simulink model "Chapter_9_Section_6_Model"  (R2019b)
settings: Solver=FixedStepAuto  StartTime=0.0  StopTime=500  FixedStep=0.02  RelTol=1e-3  EnableMultiTasking=on
libraries: arduinolib x1, simulink x1
settings Model: SimulationMode=external  ExtModeTrigDuration=2  Creator=nbibin001  LastModifiedBy=covasanvictor
settings DataIOCC: ReturnWorkspaceOutputs=off
settings OptimizationCC: PassReuseOutputArgsAs=Individual arguments  MaxStackSize=64  EfficientTunableParamExpr=on
settings DebuggingCC: ParameterTunabilityLossMsg=error  ArithmeticOperatorsInVariantConditions=warning
settings HardwareCC: ProdBitPerInt=16  ProdBitPerPointer=16  ProdBitPerSizeT=16  ProdBitPerPtrDiffT=16  ProdLargestAtomicFloat=None  ProdWordSize=8  ProdHWDeviceType=Atmel->AVR
settings SFSimCC: SimUseLocalCustomCode=off  MATLABDynamicMemAlloc=off  CustomCodeUndefinedFunction=UseInterfaceOnly
settings RTWCC: SystemTargetFile=ert.tlc  HardwareBoard=Arduino Mega 2560  TLCOptions=-aInlineSetEventsForThisBaseRateFcn=TLC_FALSE -aSuppressMultiTaskScheduler=TLC_FALSE -aRateBasedStepFcn=1  TemplateMakefile=ert_default_tmf  GenerateReport=on  RTWUseLocalCustomCode=off  Toolchain=Arduino AVR  BuildConfiguration=Faster Runs  IncludeHyperlinkInReport=on  LaunchReport=on  GenerateTraceInfo=on  GenerateTraceReport=on  GenerateTraceReportSl=on  GenerateTraceReportSf=on  GenerateTraceReportEml=on
settings CodeAppCC: ForceParamTrailComments=on  IgnoreCustomStorageClasses=off  OperatorAnnotations=on  SimulinkDataObjDesc=on  SFDataObjDesc=on  MATLABFcnDesc=on  InsertBlockDesc=on  StateflowObjectComments=on  MATLABSourceComments=on
settings ERTTargetCC: SupportContinuousTime=on  SupportVariableSizeSignals=on

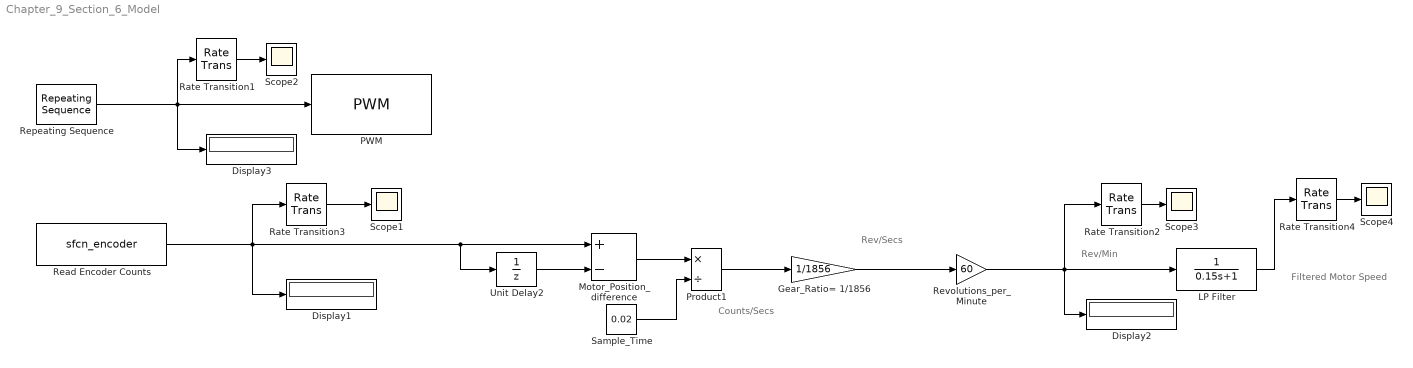
== system Chapter_9_Section_6_Model ==
  note: Counts/Secs
  note: Rev/Secs
  note: Rev/Min
  note: Filtered Motor Speed
  Display1 : Display
  Display2 : Display
  Display3 : Display
  Gear_Ratio= 1/1856 : Gain  Gain=1/1856
  LP Filter : TransferFcn  Denominator=[0.15 1]
  Motor_Position_difference : Sum  Inputs=+-
  PWM : arduinolib/PWM  pinNumber=5  EnableInputFrequency=off  InitialFrequency=2000  InitialDutyCycle=0  NotificationType=None  blockPlatform=arduino
  Product1 : Product  Inputs=*/
  Rate Transition{1..4} (4 alike) : RateTransition
  Read Encoder Counts : S-Function  InitFcn=try, set_param(gcb,'FunctionName','sfcn_encoder'), end  FunctionName=sfcn_encoder  Parameters=uint8(0),uint8(2),uint8(3)  SFunctionModules=sfcn_encoder_wrapper  SFunctionDeploymentMode=off  EnableBusSupport=off  mask(S-Function Builder){}
      mask init:
      | val = [[.9  0.75 0.75 1 1 .9 .9 1]',[1 1 0.75 0.75 .9 .9 1 .9]'];try , sys = get_param(gcb,'SfunBuilderFcnName');if isempty(sys), sys = get_param(gcb,'FunctionName'); end,catch, sys = get_param(gcb,'FunctionName'); end
      settings: CopyFcn=set_param(gcbh,'LinkStatus','none')  PreSaveFcn=try, set_param(gcb,'FunctionName','sfcn_encoder'), end  OpenFcn=sfunctionwizard(gcbh)
      mask Display: plot(val(:,1),val(:,2)),disp(sys), port_label('output',1,'pos')
  Repeating Sequence : simulink/Sources/Repeating Sequence  rep_seq_t="[0 \t  49.9   50   99.9 100  149.9  150 199.9 \t200   249.9   250 299.9 300   349.9   350 399.9 400   449.9   450 500]"  rep_seq_y="[25.5 25.5   50.1 50.1 76.5 76.5   102 102\t    127.5 127.5   153 153   178.5 178.5   204 204   229.5 229.5   255 255]"
  Revolutions_per_Minute : Gain  Gain=60
  Sample_Time : Constant  Value=0.02
  Scope{1..4} (4 alike) : Scope
  Unit Delay2 : UnitDelay  SampleTime=-1  HasFrameUpgradeWarning=on
  wires:
  Repeating Sequence/1 -> PWM/1, Rate Transition1/1, Display3/1
  Unit Delay2/1 -> Motor_Position_difference/2
  Sample_Time/1 -> Product1/2
  Product1/1 -> Gear_Ratio= 1/1856/1
  Gear_Ratio= 1/1856/1 -> Revolutions_per_Minute/1
  Revolutions_per_Minute/1 -> LP Filter/1, Display2/1, Rate Transition2/1
  Motor_Position_difference/1 -> Product1/1
  Rate Transition2/1 -> Scope3/1
  Rate Transition1/1 -> Scope2/1
  Rate Transition3/1 -> Scope1/1
  Read Encoder Counts/1 -> Display1/1, Rate Transition3/1, Motor_Position_difference/1, Unit Delay2/1
  LP Filter/1 -> Rate Transition4/1
  Rate Transition4/1 -> Scope4/1
